simulink model "factorial"  (R2021b)
settings: Solver=FixedStepDiscrete  StartTime=0.0  StopTime=10.0  RelTol=1e-3  EnableMultiTasking=on
settings Model: Creator=midol  LastModifiedBy=midol
settings DataIOCC: ReturnWorkspaceOutputs=off
settings OptimizationCC: DefaultParameterBehavior=Inlined  InlineInvariantSignals=on  EnableMemcpy=off  LifeSpan=1  EfficientTunableParamExpr=on
settings DebuggingCC: UnderspecifiedInitializationDetection=Classic  MergeDetectMultiDrivingBlocksExec=none  SFMachineParentedDataDiag=warning  ArithmeticOperatorsInVariantConditions=warning
settings ModelReferenceCC: PropagateSignalLabelsOutOfModel=off
settings SFSimCC: MATLABDynamicMemAlloc=off  CustomCodeUndefinedFunction=UseInterfaceOnly
settings RTWCC: Description=Embedded Coder  SystemTargetFile=ert.tlc  GenCodeOnly=on  TemplateMakefile=ert_default_tmf  GenerateReport=on  IncludeHyperlinkInReport=on  LaunchReport=on  GenerateTraceInfo=on  GenerateTraceReport=on  GenerateTraceReportSl=on  GenerateTraceReportSf=on  GenerateTraceReportEml=on
settings CodeAppCC: ForceParamTrailComments=on  IgnoreCustomStorageClasses=off  OperatorAnnotations=on  SimulinkDataObjDesc=on  SFDataObjDesc=on  MATLABFcnDesc=on  InsertBlockDesc=on  StateflowObjectComments=on  MATLABSourceComments=on
settings ERTTargetCC: MultiwordLength=2048  GenerateSampleERTMain=on  InlinedParameterPlacement=NonHierarchical  ERTCustomFileTemplate=example_file_process.tlc

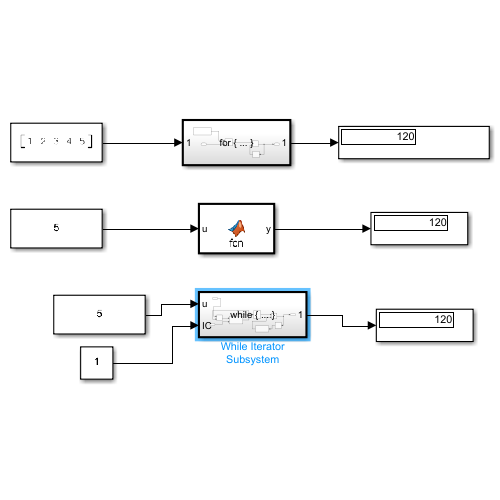
[thumbnail: Simulink's stored preview of the top-level diagram]
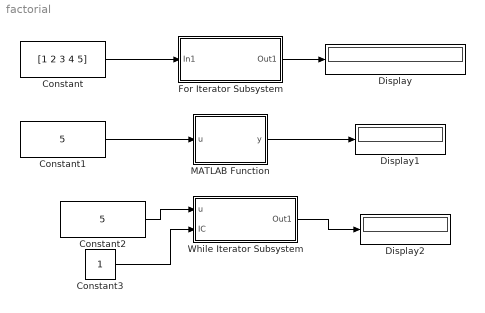
== system factorial ==
  Constant : Constant  Value=[1 2 3 4 5]
  Constant1 : Constant  Value=5
  Constant2 : Constant  Value=5
  Constant3 : Constant
  Display : Display
  Display1 : Display
  Display2 : Display
  For Iterator Subsystem : Subsystem  TreatAsAtomicUnit=on
  MATLAB Function : MATLAB Function  TreatAsAtomicUnit=on
  While Iterator Subsystem : Subsystem  TreatAsAtomicUnit=on
  wires:
  Constant/1 -> For Iterator Subsystem/1(In1)
  For Iterator Subsystem/1(Out1) -> Display/1
  Constant1/1 -> MATLAB Function/1(u)
  MATLAB Function/1(y) -> Display1/1
  Constant3/1 -> While Iterator Subsystem/2(IC)
  While Iterator Subsystem/1(Out1) -> Display2/1
  Constant2/1 -> While Iterator Subsystem/1(u)

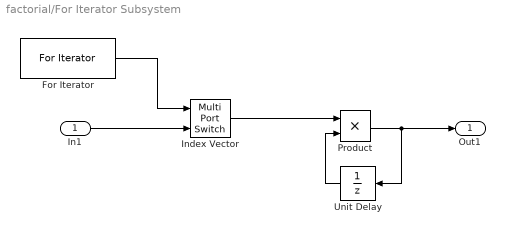
== system factorial/For Iterator Subsystem ==
  In1 : Inport
  For Iterator : ForIterator  ResetStates=reset  IndexMode=Zero-based
  Index Vector : MultiPortSwitch  DataPortOrder=Zero-based contiguous  Inputs=1  zeroidx=on
  Product : Product
  Unit Delay : UnitDelay  InitialCondition=1  SampleTime=-1  HasFrameUpgradeWarning=on
  Out1 : Outport
  wires:
  For Iterator/1 -> Index Vector/1
  In1/1 -> Index Vector/2
  Index Vector/1 -> Product/1
  Product/1 -> Unit Delay/1, Out1/1
  Unit Delay/1 -> Product/2

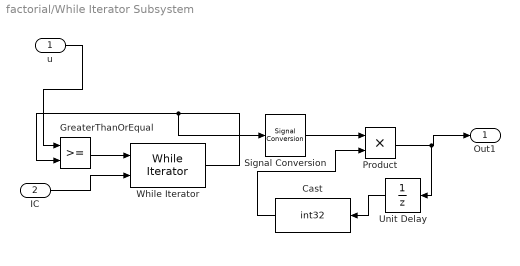
== system factorial/While Iterator Subsystem ==
  u : Inport
  IC : Inport  Port=2
  Cast : DataTypeConversion  OutDataTypeStr=int32
  GreaterThanOrEqual : RelationalOperator  OutDataTypeStr=boolean  RndMeth=Simplest
  Product : Product
  Signal Conversion : SignalConversion  OverrideOpt=off
  Unit Delay : UnitDelay  InitialCondition=1  SampleTime=-1  HasFrameUpgradeWarning=on
  While Iterator : WhileIterator  ResetStates=reset  ShowIterationPort=on
  Out1 : Outport
  wires:
  IC/1 -> While Iterator/2
  u/1 -> GreaterThanOrEqual/1
  GreaterThanOrEqual/1 -> While Iterator/1
  Product/1 -> Unit Delay/1, Out1/1
  While Iterator/1 -> GreaterThanOrEqual/2, Signal Conversion/1
  Signal Conversion/1 -> Product/1
  Unit Delay/1 -> Cast/1
  Cast/1 -> Product/2

== matlab function factorial/MATLAB Function ==
  data: u input; y output
function y = fcn(u)

    if u > 0
        y = factorial(u);
    else
        y = 0;
    end
